simulink model "scheme4"  (R2022b)
settings: Solver=VariableStepAuto  StartTime=0.0  StopTime=15  MaxStep=0.01  RelTol=1e-3
libraries: simulink x4
settings Model: Creator=alyok  LastModifiedBy=alyok

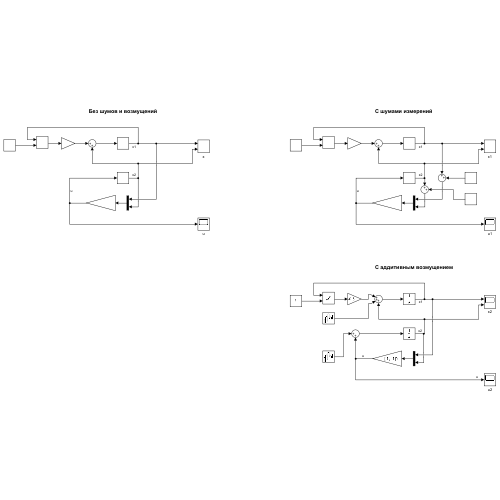
[thumbnail: Simulink's stored preview of the top-level diagram]
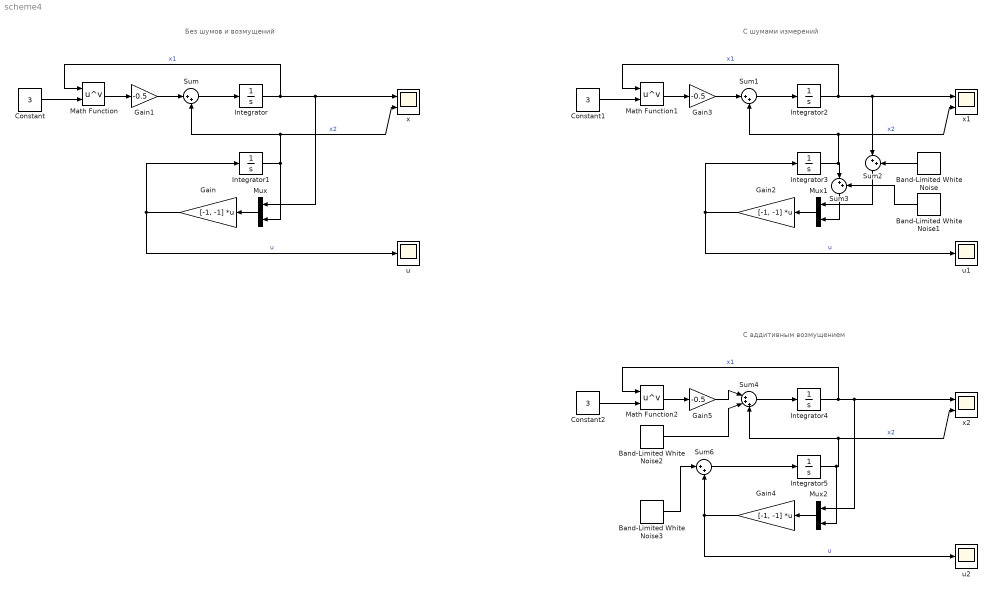
== system scheme4 ==
  note: Без шумов и возмущений
  note: С шумами измерений
  note: С аддитивным возмущением
  Band-Limited White Noise{,1..3} (4 alike) : simulink/Sources/Band-Limited White Noise  Cov=[0.0001]  Ts=0.01  seed=[23341]
  Constant : Constant  Value=3
  Constant1 : Constant  Value=3
  Constant2 : Constant  Value=3
  Gain : Gain  Gain=[-1, -1]  Multiplication=Matrix(K*u)
  Gain1 : Gain  Gain=-0.5
  Gain2 : Gain  Gain=[-1, -1]  Multiplication=Matrix(K*u)
  Gain3 : Gain  Gain=-0.5
  Gain4 : Gain  Gain=[-1, -1]  Multiplication=Matrix(K*u)
  Gain5 : Gain  Gain=-0.5
  Integrator{,1..5} (6 alike) : Integrator  InitialCondition=1
  Math Function : Math  Operator=pow
  Math Function1 : Math  Operator=pow
  Math Function2 : Math  Operator=pow
  Mux : Mux  Inputs=2
  Mux1 : Mux  Inputs=2
  Mux2 : Mux  Inputs=2
  Sum{,1..3,6} (5 alike) : Sum  Inputs=|++
  Sum4 : Sum  Inputs=|+++
  u : Scope
  u1 : Scope
  u2 : Scope
  x : Scope  NumInputPorts=2
  x1 : Scope  NumInputPorts=2
  x2 : Scope  NumInputPorts=2
  wires:
  Sum/1 -> Integrator/1
  Integrator1/1 -> Sum/2, x/2, Mux/2  "x2"
  Gain/1 -> Integrator1/1, u/1  "u"
  Math Function/1 -> Gain1/1
  Integrator/1 -> Mux/1, x/1, Math Function/1  "x1"
  Constant/1 -> Math Function/2
  Gain1/1 -> Sum/1
  Mux/1 -> Gain/1
  Constant1/1 -> Math Function1/2
  Gain3/1 -> Sum1/1
  Mux1/1 -> Gain2/1
  Math Function1/1 -> Gain3/1
  Gain2/1 -> Integrator3/1, u1/1  "u"
  Integrator2/1 -> x1/1, Sum2/1, Math Function1/1  "x1"
  Sum1/1 -> Integrator2/1
  Integrator3/1 -> Sum3/1, Sum1/2, x1/2  "x2"
  Band-Limited White Noise/1 -> Sum2/2
  Sum2/1 -> Mux1/1
  Sum3/1 -> Mux1/2
  Band-Limited White Noise1/1 -> Sum3/2
  Integrator4/1 -> Mux2/1, x2/1, Math Function2/1  "x1"
  Band-Limited White Noise3/1 -> Sum6/1
  Band-Limited White Noise2/1 -> Sum4/2
  Gain4/1 -> u2/1, Sum6/2  "u"
  Math Function2/1 -> Gain5/1
  Gain5/1 -> Sum4/1
  Mux2/1 -> Gain4/1
  Constant2/1 -> Math Function2/2
  Integrator5/1 -> Mux2/2, Sum4/3, x2/2  "x2"
  Sum4/1 -> Integrator4/1
  Sum6/1 -> Integrator5/1
